simulink model "KMS"  (R2024a)
settings: Solver=FixedStepDiscrete  StartTime=0.0  StopTime=inf  FixedStep=param.t_sample  RelTol=1e-3
undefined symbols (not defined in the file): param
settings Model: SimulationMode=external  ExtModeTrigDuration=10000  ExtModeArchiveMode=auto  ExtModeArchiveFileName=measurement_data  ExtModeArchiveDirName=/home/pkr_devpc/Schreibtisch/Git/3rrr_pkm/Versuchsstand/result  ExtModeLogAll=off  Creator=schappler  LastModifiedBy=mohammad_admin
settings SolverCC: AlgebraicLoopSolver=TrustRegion  MinimalZcImpactIntegration=on
settings DataIOCC: SaveOutput=off  SignalLogging=off  SaveTime=off  ReturnWorkspaceOutputs=off
settings OptimizationCC: BufferReuse=off  GlobalBufferReuse=off  ExpressionFolding=off  LocalBlockOutputs=off  OptimizeDataStoreBuffers=off  BusAssignmentInplaceUpdate=off
settings DebuggingCC: ReadBeforeWriteMsg=DisableAll  WriteAfterWriteMsg=DisableAll  WriteAfterReadMsg=DisableAll  MultiTaskDSMMsg=none  UnconnectedInputMsg=warning  UnconnectedOutputMsg=warning  UnconnectedLineMsg=warning  ArithmeticOperatorsInVariantConditions=warning
settings ModelReferenceCC: UpdateModelReferenceTargets=IfOutOfDate  EnableRefExpFcnMdlSchedulingChecks=on
settings SFSimCC: SFSimEcho=off  CustomCodeUndefinedFunction=UseInterfaceOnly
settings RTWCC: Description=EtherLab PREEMT_RT Real-Time Target  SystemTargetFile=etherlab.tlc  TemplateMakefile=etherlab_hrt.tmf  GenerateReport=on  LaunchReport=on  GPUComputeCapability=3.5
settings STFCustomTargetCC: UseToolchainInfoCompliant=off  SystemTargetFile=etherlab.tlc
settings GRTTargetCC: ParMdlRefBuildCompliant=off  CompOptLevelCompliant=off  ConcurrentExecutionCompliant=off  CombineOutputUpdateFcns=off  MatFileLogging=off  CPPClassGenCompliant=off  GRTInterface=on  UseToolchainInfoCompliant=off  ExtMode=on  ExtModeStaticAlloc=on  ExtModeStaticAllocSize=2000000000  ExtModeMexArgs='10.144.130.139' 0 17725  RTWCAPISignals=on  RTWCAPIParams=on

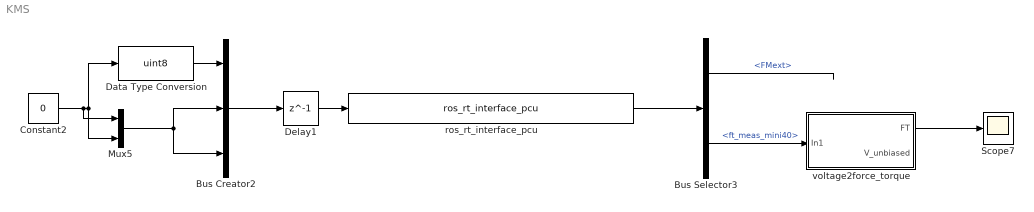
== system KMS ==
  Bus Creator2 : BusCreator  Inputs=3
  Bus Selector3 : BusSelector  OutputSignals=FMext,ft_meas_mini40
  Constant2 : Constant  Value=0  SampleTime=-1
  Data Type Conversion : DataTypeConversion  OutDataTypeStr=uint8  SaturateOnIntegerOverflow=off  RndMeth=Floor
  Delay1 : Delay  DelayLength=1
  Mux5 : Mux  Inputs=2
  Scope7 : Scope
  ros_rt_interface_pcu : S-Function  FunctionName=ros_rt_interface_pcu  SFunctionDeploymentMode=off  EnableBusSupport=off  mask(Legacy Function){SFunctionSpec=void SL_io_func(SL_OUT_type u1[1], SL_IN_type y1[1]), ShowSpec=on}
      mask prompts: ShowSpec "Display function specification"
      mask help:
      | This block allows you to call the legacy functions specified by the following Legacy Code Tool definition:
      | def.SFunctionName = 'ros_rt_interface_pcu';
      | def.OutputFcnSpec = 'void SL_io_func(SL_OUT_type u1[1], SL_IN_type y1[1])';
      | def.StartFcnSpec = 'void SL_start_func()';
      | def.TerminateFcnSpec = 'void SL_terminate_func()';
      | def.HeaderFiles = {'SL_func.h'};
      | def.SourceFiles = {'../ros_rt_interface/ros_rt_core/SL_func_dummy.cpp'};
      | def.TargetLibFiles = {'libros_sl_interface.so'};
      | def.IncPaths = {'../ros_rt_interface/ros_rt_core'};
      mask Help: <p>This block was generated automatically by the Legacy Code Tool. For detailed help on this tool, call<a href="matlab:legacy_code('help')"> legacy_code('help')</a>.</p>
      mask Callback ShowSpec:
      | if strcmp(get_param(gcbh, 'ShowSpec'), 'on')
      |   set_param(gcbh, 'MaskDisplay', sprintf('fprintf(''%s'');', get_param(gcbh, 'SFunctionSpec')));
      | else
      |   set_param(gcbh, 'MaskDisplay', sprintf('fprintf(''%s'');', get_param(gcbh, 'FunctionName')));
      | end
      mask Display: fprintf('void SL_io_func(SL_OUT_type u1[1], SL_IN_type y1[1])');
  voltage2force_torque : Subsystem
  wires:
  Bus Creator2/1 -> Delay1/1
  Data Type Conversion/1 -> Bus Creator2/1
  Bus Selector3/2 -> voltage2force_torque/1(In1)  "<ft_meas_mini40>"
  Bus Selector3/1 -> ?  "<FMext>"
  Mux5/1 -> Bus Creator2/3, Bus Creator2/2
  voltage2force_torque/1(FT) -> Scope7/1
  ros_rt_interface_pcu/1 -> Bus Selector3/1
  Delay1/1 -> ros_rt_interface_pcu/1
  Constant2/1 -> Mux5/2, Data Type Conversion/1, Mux5/1

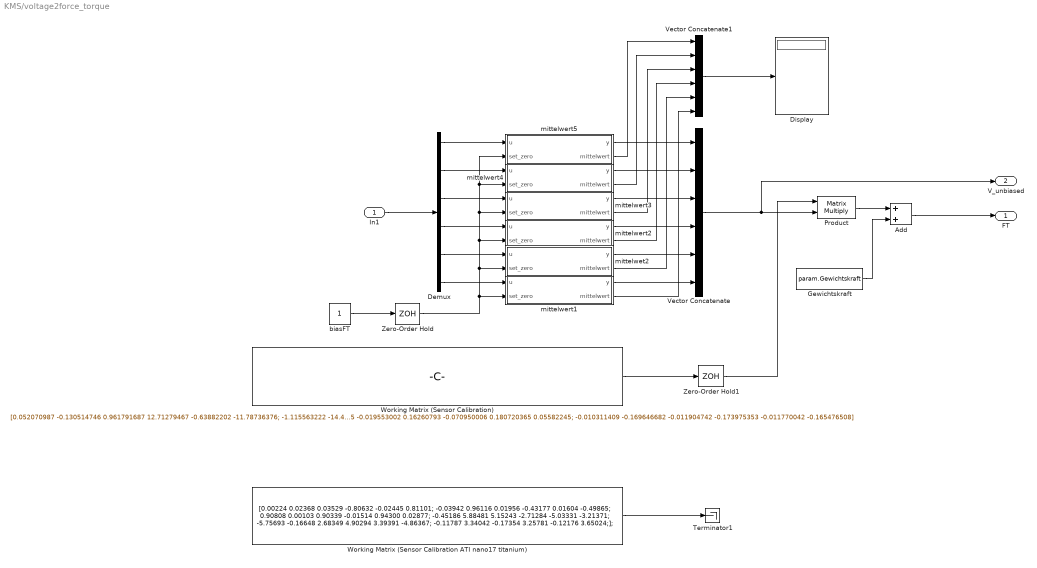
== system KMS/voltage2force_torque ==
  In1 : Inport
  Add : Sum
  Demux : Demux  Outputs=6
  Display : Display
  Gewichtskraft : Constant  Value=param.Gewichtskraft  SampleTime=-1
  Product : Product  Multiplication=Matrix(*)  RndMeth=Zero
  Terminator1 : Terminator
  Vector Concatenate : Concatenate  NumInputs=6  Mode=Multidimensional array
  Vector Concatenate1 : Concatenate  NumInputs=6  Mode=Multidimensional array
  Working Matrix (Sensor Calibration ATI nano17 titanium) : Constant  Value=|  SampleTime=-1
      | [0.00224   0.02368   0.03529  -0.80632  -0.02445   0.81101;
      |     -0.03942   0.96116   0.01956  -0.43177   0.01604  -0.49865;
      | 	0.90808   0.00103   0.90339  -0.01514   0.94300   0.02877;
      | 	-0.45186   5.88481   5.15243  -2.71284  -5.03331  -3.21371;
      | 	-5.75693  -0.16648   2.68349   4.90294   3.39391  -4.86367;
      | 	-0.11787   3.34042  -0.17354   3.25781  -0.12176   3.65024;];
  Working Matrix (Sensor Calibration) : Constant  Value=|  SampleTime=-1
      | [0.052070987 -0.130514746 0.961791687 12.71279467 -0.63882202 -11.78736376;
      | -1.115563222 -14.4308958 0.66281852 7.178188359 0.390451919 7.011768932;
      | 21.03335044 1.08132865 20.50422466 -0.287397369 21.07979804 -1.27937419;
      | -0.012415733 -0.080850353 0.29706849 0.038847671 -0.303166527 0.053776337;
      | -0.337109545 -0.019553002 0.16260793 -0.070950006 0.180720365 0.05582245;
      | -0.010311409 -0.169646682 -0.011904742 -0.173975353 -0.011770042 -0.165476508]
  Zero-Order Hold : ZeroOrderHold  SampleTime=-1
  Zero-Order Hold1 : ZeroOrderHold  SampleTime=-1
  biasFT : Constant  SampleTime=-1
  mittelwert1 : MATLAB Function  TreatAsAtomicUnit=on
  mittelwert2 : MATLAB Function  TreatAsAtomicUnit=on
  mittelwert3 : MATLAB Function  TreatAsAtomicUnit=on
  mittelwert4 : MATLAB Function  TreatAsAtomicUnit=on
  mittelwert5 : MATLAB Function  TreatAsAtomicUnit=on
  mittelwet2 : MATLAB Function  TreatAsAtomicUnit=on
  FT : Outport  VectorParamsAs1DForOutWhenUnconnected=off
  V_unbiased : Outport  Port=2  VectorParamsAs1DForOutWhenUnconnected=off
  wires:
  Demux/2 -> mittelwert4/1(u)
  mittelwert2/2(mittelwert) -> Vector Concatenate1/4
  Demux/3 -> mittelwert3/1(u)
  Demux/5 -> mittelwet2/1(u)
  mittelwert1/1(y) -> Vector Concatenate/6
  mittelwert3/2(mittelwert) -> Vector Concatenate1/3
  mittelwert2/1(y) -> Vector Concatenate/4
  mittelwert5/2(mittelwert) -> Vector Concatenate1/1
  mittelwert5/1(y) -> Vector Concatenate/1
  mittelwert3/1(y) -> Vector Concatenate/3
  mittelwert4/1(y) -> Vector Concatenate/2
  Demux/6 -> mittelwert1/1(u)
  Demux/4 -> mittelwert2/1(u)
  mittelwet2/1(y) -> Vector Concatenate/5
  Demux/1 -> mittelwert5/1(u)
  In1/1 -> Demux/1
  mittelwert1/2(mittelwert) -> Vector Concatenate1/6
  mittelwert4/2(mittelwert) -> Vector Concatenate1/2
  mittelwet2/2(mittelwert) -> Vector Concatenate1/5
  Zero-Order Hold/1 -> mittelwert1/2(set_zero), mittelwet2/2(set_zero), mittelwert2/2(set_zero), mittelwert3/2(set_zero), mittelwert4/2(set_zero), mittelwert5/2(set_zero)
  Zero-Order Hold1/1 -> Product/1
  Vector Concatenate/1 -> V_unbiased/1, Product/2
  Vector Concatenate1/1 -> Display/1
  Product/1 -> Add/1
  Add/1 -> FT/1
  biasFT/1 -> Zero-Order Hold/1
  Gewichtskraft/1 -> Add/2
  Working Matrix (Sensor Calibration)/1 -> Zero-Order Hold1/1
  Working Matrix (Sensor Calibration ATI nano17 titanium)/1 -> Terminator1/1

== matlab function KMS/voltage2force_torque/mittelwert2 ==
  data: u input; y output; set_zero input; mittelwert output
function [y,mittelwert] = mittelwert(u, set_zero)
%#eml
persistent zustand;
persistent mittelwert_z;
persistent i;
if isempty(zustand)
    zustand = 0.0;
    i=1;
    mittelwert_z = 0.0;
end;

if set_zero == 1 && zustand == 0
    zustand = 1;
    mittelwert_z = 0.0;
    i = 1;
elseif set_zero == 0 
    zustand = 0;
end;
    
if zustand == 1
        mittelwert_z = (mittelwert_z * (i-1) + u)/i;
        i=i+1;
end;

y = u - mittelwert_z;
mittelwert = mittelwert_z;

== matlab function KMS/voltage2force_torque/mittelwert3 ==
  data: u input; y output; set_zero input; mittelwert output
function [y,mittelwert] = mittelwert(u, set_zero)
%#eml
persistent zustand;
persistent mittelwert_z;
persistent i;
if isempty(zustand)
    zustand = 0.0;
    i=1;
    mittelwert_z = 0.0;
end;

if set_zero == 1 && zustand == 0
    zustand = 1;
    mittelwert_z = 0.0;
    i = 1;
elseif set_zero == 0 
    zustand = 0;
end;
    
if zustand == 1
        mittelwert_z = (mittelwert_z * (i-1) + u)/i;
        i=i+1;
end;

y = u - mittelwert_z;
mittelwert = mittelwert_z;

== matlab function KMS/voltage2force_torque/mittelwert4 ==
  data: u input; y output; set_zero input; mittelwert output
function [y,mittelwert] = mittelwert(u, set_zero)
%#eml
persistent zustand;
persistent mittelwert_z;
persistent i;
if isempty(zustand)
    zustand = 0.0;
    i=1;
    mittelwert_z = 0.0;
end;

if set_zero == 1 && zustand == 0
    zustand = 1;
    mittelwert_z = 0.0;
    i = 1;
elseif set_zero == 0 
    zustand = 0;
end;
    
if zustand == 1
        mittelwert_z = (mittelwert_z * (i-1) + u)/i;
        i=i+1;
end;

y = u - mittelwert_z;
mittelwert = mittelwert_z;

== matlab function KMS/voltage2force_torque/mittelwert5 ==
  data: u input; y output; set_zero input; mittelwert output
function [y,mittelwert] = mittelwert(u, set_zero)
%#codegen
persistent zustand;
persistent mittelwert_z;
persistent i;
if isempty(zustand)
    zustand = 0.0;
    i=1;
    mittelwert_z = 0.0;
end;

if set_zero == 1 && zustand == 0
    zustand = 1;
    mittelwert_z = 0.0;
    i = 1;
elseif set_zero == 0 
    zustand = 0;
end;
    
if zustand == 1
        mittelwert_z = (mittelwert_z * (i-1) + u)/i;
        i=i+1;
end;

y = u - mittelwert_z;
mittelwert = mittelwert_z;

== matlab function KMS/voltage2force_torque/mittelwet2 ==
  data: u input; y output; set_zero input; mittelwert output
function [y,mittelwert] = mittelwert(u, set_zero)
%#eml
persistent zustand;
persistent mittelwert_z;
persistent i;
if isempty(zustand)
    zustand = 0.0;
    i=1;
    mittelwert_z = 0.0;
end;

if set_zero == 1 && zustand == 0
    zustand = 1;
    mittelwert_z = 0.0;
    i = 1;
elseif set_zero == 0 
    zustand = 0;
end;
    
if zustand == 1
        mittelwert_z = (mittelwert_z * (i-1) + u)/i;
        i=i+1;
end;

y = u - mittelwert_z;
mittelwert = mittelwert_z;

== matlab function KMS/voltage2force_torque/mittelwert1 ==
  data: u input; y output; set_zero input; mittelwert output
function [y,mittelwert] = mittelwert(u, set_zero)
%#eml
persistent zustand;
persistent mittelwert_z;
persistent i;
if isempty(zustand)
    zustand = 0.0;
    i=1;
    mittelwert_z = 0.0;
end;

if set_zero == 1 && zustand == 0
    zustand = 1;
    mittelwert_z = 0.0;
    i = 1;
elseif set_zero == 0 
    zustand = 0;
end;
    
if zustand == 1
        mittelwert_z = (mittelwert_z * (i-1) + u)/i;
        i=i+1;
end;

y = u - mittelwert_z;
mittelwert = mittelwert_z;
